simulink model "Automated_Headlamps"  (R2025a)
settings: Solver=FixedStepAuto  StartTime=0.0  StopTime=70  RelTol=1e-3
libraries: simulink x3
settings Model: Creator=Rudransh  LastModifiedBy=Rudransh
settings OptimizationCC: DefaultParameterBehavior=Inlined  EnhancedBackFolding=on  PassReuseOutputArgsAs=Individual arguments  ZeroExternalMemoryAtStartup=off  ZeroInternalMemoryAtStartup=off  OptimizeBlockOrder=speed  DifferentSizesBufferReuse=on  OptimizationCustomize=off  EfficientTunableParamExpr=on
settings DebuggingCC: ParameterTunabilityLossMsg=error
settings SFSimCC: MATLABDynamicMemAlloc=off
settings RTWCC: SystemTargetFile=ert.tlc  TemplateMakefile=ert_default_tmf  DataTypeReplacement=CDataTypesFixedWidth  Description=Embedded Coder
settings CodeAppCC: ForceParamTrailComments=on  IgnoreCustomStorageClasses=off  OperatorAnnotations=on  SimulinkDataObjDesc=on  SFDataObjDesc=on  InsertBlockDesc=on
settings ERTTargetCC: ExtModeTransport=0.0  ExtModeStaticAlloc=off  ExtModeMexFile=ext_comm  ExtModeIntrfLevel=Level1  ERTCustomFileTemplate=example_file_process.tlc  MaxIdInt64=INT64_MAX  MinIdInt64=INT64_MIN  MaxIdUint64=UINT64_MAX  MaxIdInt32=INT32_MAX  MinIdInt32=INT32_MIN  MaxIdUint32=UINT32_MAX  MaxIdInt16=INT16_MAX  MinIdInt16=INT16_MIN  MaxIdUint16=UINT16_MAX  MaxIdInt8=INT8_MAX  MinIdInt8=INT8_MIN  MaxIdUint8=UINT8_MAX  TargetLangStandard=C99 (ISO)  GenerateSampleERTMain=on

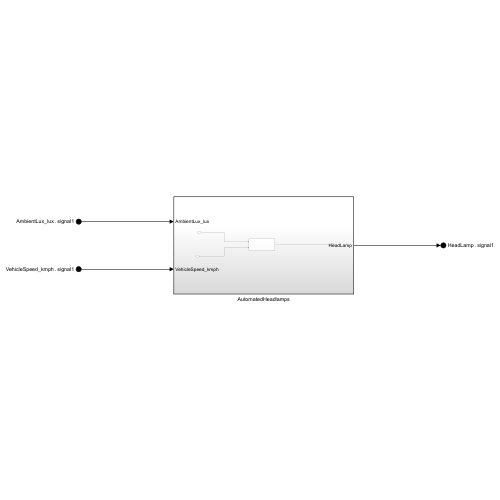
[thumbnail: Simulink's stored preview of the top-level diagram]
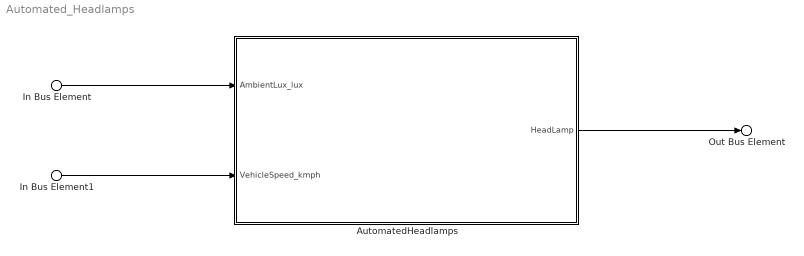
== system Automated_Headlamps ==
  In Bus Element : Inport  PortName=AmbientLux_lux  Element=signal1
  In Bus Element1 : Inport  Port=2  PortName=VehicleSpeed_kmph  Element=signal1
  AutomatedHeadlamps : Subsystem
  Out Bus Element : Outport  PortName=HeadLamp  Element=signal1
  wires:
  In Bus Element1/1 -> AutomatedHeadlamps/2(VehicleSpeed_kmph)
  In Bus Element/1 -> AutomatedHeadlamps/1(AmbientLux_lux)
  AutomatedHeadlamps/1(HeadLamp) -> Out Bus Element/1

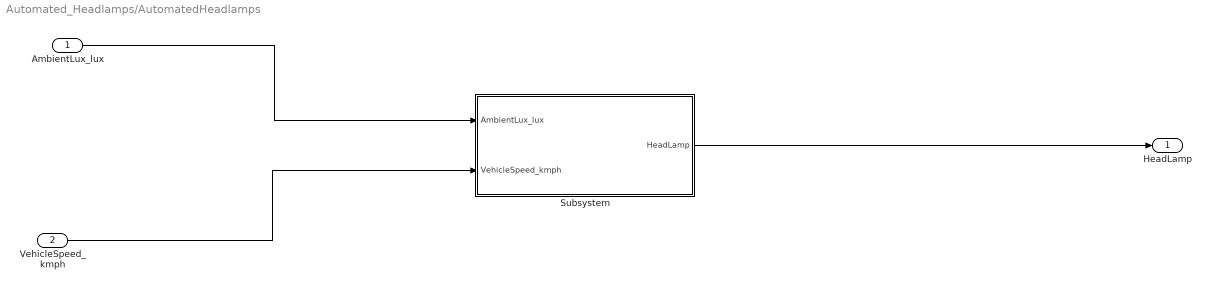
== system Automated_Headlamps/AutomatedHeadlamps ==
  AmbientLux_lux : Inport
  VehicleSpeed_kmph : Inport  Port=2
  Subsystem : Subsystem
  HeadLamp : Outport
  wires:
  Subsystem/1(HeadLamp) -> HeadLamp/1
  VehicleSpeed_kmph/1 -> Subsystem/2(VehicleSpeed_kmph)
  AmbientLux_lux/1 -> Subsystem/1(AmbientLux_lux)

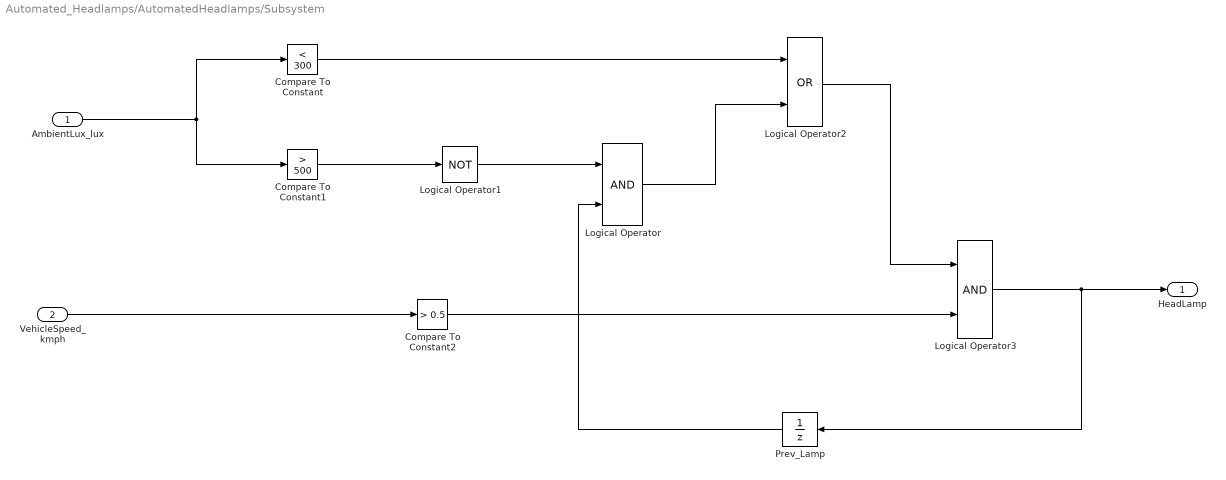
== system Automated_Headlamps/AutomatedHeadlamps/Subsystem ==
  AmbientLux_lux : Inport
  VehicleSpeed_kmph : Inport  Port=2
  Compare To Constant : simulink/Logic and Bit Operations/Compare To Constant  relop=<  const=300  OutDataTypeStr=boolean
  Compare To Constant1 : simulink/Logic and Bit Operations/Compare To Constant  relop=>  const=500  OutDataTypeStr=boolean
  Compare To Constant2 : simulink/Logic and Bit Operations/Compare To Constant  relop=>  const=0.5  OutDataTypeStr=boolean
  Logical Operator : Logic  AllPortsSameDT=off  OutDataTypeStr=boolean
  Logical Operator1 : Logic  Operator=NOT  AllPortsSameDT=off  OutDataTypeStr=boolean
  Logical Operator2 : Logic  Operator=OR  AllPortsSameDT=off  OutDataTypeStr=boolean
  Logical Operator3 : Logic  AllPortsSameDT=off  OutDataTypeStr=boolean
  Prev_Lamp : UnitDelay  SampleTime=-1  HasFrameUpgradeWarning=on
  HeadLamp : Outport
  wires:
  Logical Operator3/1 -> HeadLamp/1, Prev_Lamp/1
  Compare To Constant1/1 -> Logical Operator1/1
  AmbientLux_lux/1 -> Compare To Constant/1, Compare To Constant1/1
  Logical Operator/1 -> Logical Operator2/2
  Prev_Lamp/1 -> Logical Operator/2
  Logical Operator1/1 -> Logical Operator/1
  Compare To Constant/1 -> Logical Operator2/1
  VehicleSpeed_kmph/1 -> Compare To Constant2/1
  Compare To Constant2/1 -> Logical Operator3/2
  Logical Operator2/1 -> Logical Operator3/1
